simulink model "extra_blocks"  (Simulink 7.4)
settings: Solver=FixedStepDiscrete  StartTime=0.0  StopTime=10.0  RelTol=1e-3
undefined symbols (not defined in the file or in its folder): Ax, Ay, Az, DiscIntNeverNeededParam, lenA, sys1d, vargz
libraries: simulink x8, dspsigops x1, commanapbnd3 x1, instrumentlib x1
(part 1 of 2)
settings Model: Creator=iMose1  LastModifiedBy=iMose1

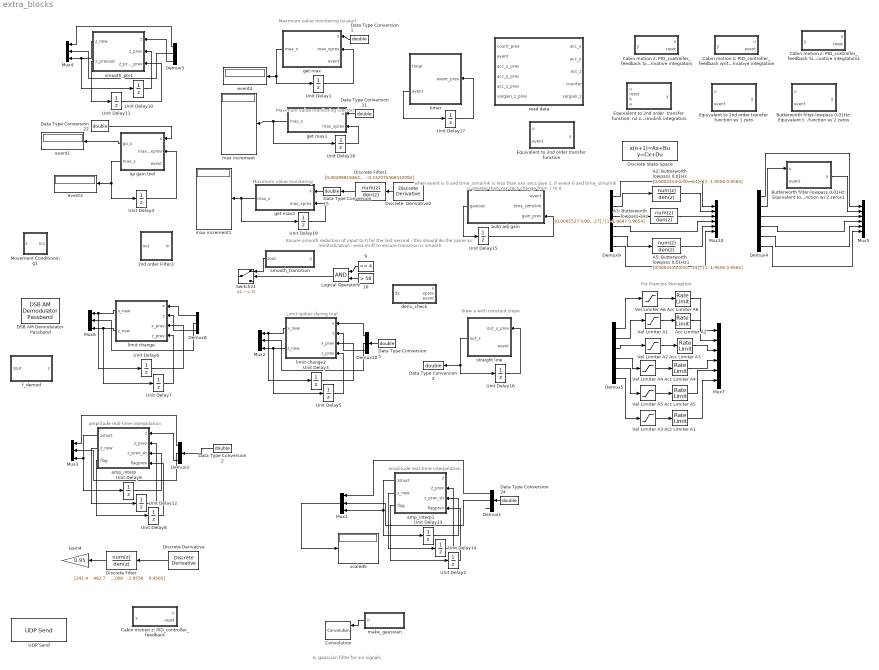
== system extra_blocks ==
  note: Limit spikes during trial
  note: amplitude real-time interpolation
  note: Ensure smooth reduction of input to 0
      | for the last second - this should do the
      | same as reinitialization - exta stuff
      | to ensure transition is smooth
  note: amplitude real-time interpolation
  note: draw a with
      | constant slope
  note: 6. gaussian filter
      | for sin signals
  note: when event is 6 and time_simulink is less than xxx secs give 1,
      | if event 6 and time_simulink is greater than xxx secs change from 1 to 0
  note: Maximum value monitoring (vector)
  note: Maximum value monitoring (scalar)
  note: Maximum value monitoring
  note: For Francois Perception
  "     10" : simulink/Logic and Bit Operations/Compare To Constant  SystemSampleTime=-1  relop=>  const=58  LogicOutDataTypeMode=uint8
  "     9" : simulink/Logic and Bit Operations/Compare To Constant  SystemSampleTime=-1  relop===  const=4  LogicOutDataTypeMode=uint8
  2nd order Filter2 : Subsystem
  A2: Butterworth lowpass 0.01Hz : DiscreteTransferFcn  Numerator=[0.0002414 0.0004827 0.0002414]  Denominator=[1 -1.9556 0.9565]  SampleTime=0.004
  A3: Butterworth lowpass 1Hz : DiscreteTransferFcn  Numerator=[0.0001527 0.0003054 0.0001527]  Denominator=[1 -1.9647 0.9654]  SampleTime=0.004
  A5: Butterworth lowpass 0.01Hz1 : DiscreteTransferFcn  Numerator=[0.0002414 0.0004827 0.0002414]  Denominator=[1 -1.9556 0.9565]  SampleTime=0.004
  Acc Limiter A1 : RateLimiter  RisingSlewLimit=0  FallingSlewLimit=0  SampleTimeMode=inherited
  Acc Limiter A2 : RateLimiter  RisingSlewLimit=0.05  FallingSlewLimit=-0.05  SampleTimeMode=inherited
  Acc Limiter A3 : RateLimiter  RisingSlewLimit=0.05  FallingSlewLimit=-0.05  SampleTimeMode=inherited
  Acc Limiter A4 : RateLimiter  RisingSlewLimit=0  FallingSlewLimit=0  SampleTimeMode=inherited
  Acc Limiter A5 : RateLimiter  RisingSlewLimit=0.05  FallingSlewLimit=-0.05  SampleTimeMode=inherited
  Acc Limiter A6 : RateLimiter  RisingSlewLimit=0  FallingSlewLimit=0  SampleTimeMode=inherited
  Butterworth filter-lowpass 0.01Hz: Equivalent to 2nd order transfer function w/ 2 zeros : Subsystem
  Butterworth filter-lowpass 0.01Hz: Equivalent to 2nd order transfer function w/ 2 zeros1 : Subsystem
  Cabin motion z: PID_controller_feedback : Subsystem
  Cabin motion z: PID_controller_feedback Simulink derivative integrators : Subsystem
  Cabin motion z: PID_controller_feedback Simulink derivative integrators1 : Subsystem
  Cabin motion z: PID_controller_feedback written derivative integration : Subsystem
  Convolution : dspsigops/Convolution  DialogController=dspDDGCreate  DialogControllerArgs=DataTag0  domain=Time  outputDataTypeStr=Inherit: Same as accumulator  outputLastDataTypeStr=Inherit: Same as accumulator  outputMin=[]  outputMax=[]  roundingMode=Floor  overflowMode=off
  DSB AM Demodulator Passband : commanapbnd3/DSB AM Demodulator Passband  SystemSampleTime=-1  Fc=0.091  Ph=0  method=Butterworth  n=4  cf=10  Rp=0.1  Rs=50  Offset=0
  Data Type Conversion{1..3,5,11,15,22,24} (8 alike) : DataTypeConversion  OutDataTypeMode=double  OutDataType=fixdt(1, 16)  OutScaling=2^0  OutDataTypeStr=double
  Demux{1..3,8,10} (5 alike) : Demux  Outputs=3
  Demux4 : Demux  Outputs=6
  Demux5 : Demux  Outputs=6
  Demux9 : Demux  Outputs=6
  Discrete  Derivative2 : simulink/Discrete/Discrete Derivative  SystemSampleTime=-1  gainval=1.0  ICPrevScaledInput=0.0  OutMin=[]  OutMax=[]  OutDataType=fixdt(1, 16)  OutScaling=2^-10  DoSatur=off
  Discrete Derivative : simulink/Discrete/Discrete Derivative  SystemSampleTime=-1  gainval=1.0  ICPrevScaledInput=0.0  OutMin=[]  OutMax=[]  OutDataType=fixdt(1, 16)  OutScaling=2^-10  DoSatur=off
  Discrete Filter : DiscreteFilter  Numerator="[241.4    482.7    241.4]"  Denominator="[1.0000   -1.9556    0.9565]"  SampleTime=0.004
  Discrete Filter1 : DiscreteFilter  Numerator="[0.002898194633721   0.008694583901164   0.008694583901164   0.002898194633721]"  Denominator="[1.000000000000000  -2.374094743709352   1.929355669091215  -0.532075368312092]"
  Discrete State-Space : DiscreteStateSpace  A=sys1d.a  B=sys1d.b  C=sys1d.c  D=sys1d.d  SampleTime=0.004
  Equivalent to 2nd order transfer function : Subsystem
  Equivalent to 2nd order transfer function w/ 1 zero : Subsystem
  "Equivalent to 2nd order  transfer function, no zeros, Simulink integrators" : Subsystem
  Gain4 : Gain  Gain=0.95  ParameterDataType=fixdt(1, 16)  ParameterScaling=2^0  OutDataType=fixdt(1, 16)  OutScaling=2^0
  Logical Operator9 : Logic  AllPortsSameDT=off  OutDataTypeMode=boolean  LogicDataType=fixdt(0, 8)  OutDataTypeStr=boolean
  Movement Conditioning1 : Subsystem
  Mux{1..4,6} (5 alike) : Mux  Inputs=3
  Mux10 : Mux  Inputs=6
  Mux5 : Mux  Inputs=6
  Mux7 : Mux  Inputs=6
  Switch21 : Switch  Criteria=u2 ~= 0  OutDataType=fixdt(1, 16)  OutScaling=2^0
  UDP Send : instrumentlib/UDP Send  DialogController=instrumentcreatedialog  DialogControllerArgs=DataTag1  Host='192.168.102.50'  Port=9800  LocalPort=-1  EnableBlockingMode=on  ByteOrder=BigEndian
  Unit Delay{1..17} (17 alike) : UnitDelay  SampleTime=-1
  Unit Delay18 : UnitDelay  X0=zeros(6,1)  SampleTime=-1
  Unit Delay19 : UnitDelay  X0=zeros(6,1)  SampleTime=-1
  Vel Limiter A1 : Saturate  UpperLimit=0.08  LowerLimit=-0.08  LinearizeAsGain=off  OutDataType=fixdt(1, 16)  OutScaling=2^0
  Vel Limiter A2 : Saturate  UpperLimit=0.05  LowerLimit=-0.05  OutDataType=fixdt(1, 16)  OutScaling=2^0
  Vel Limiter A3 : Saturate  UpperLimit=0  LowerLimit=0  OutDataType=fixdt(1, 16)  OutScaling=2^0
  Vel Limiter A4 : Saturate  UpperLimit=0  LowerLimit=0  OutDataType=fixdt(1, 16)  OutScaling=2^0
  Vel Limiter A5 : Saturate  UpperLimit=0.1  LowerLimit=-0.1  OutDataType=fixdt(1, 16)  OutScaling=2^0
  Vel Limiter A6 : Saturate  UpperLimit=0  LowerLimit=0  OutDataType=fixdt(1, 16)  OutScaling=2^0
  amp_interp : Stateflow chart
  amp_interp1 : Stateflow chart
  auto adj gain : Stateflow chart
  deriv_check : Stateflow chart
  event1 : Display
  event3 : Display
  event4 : Display
  f_demod : Stateflow chart
  get max : Stateflow chart
  get max1 : Stateflow chart
  get max2 : Stateflow chart
  limit change : Stateflow chart
  limit change2 : Stateflow chart
  make_gaussian : Stateflow chart
  max increment : Display
  max increment1 : Display
  op gain tool : Stateflow chart
  read data : Stateflow chart
  scaled5 : Display
  smooth_pts1 : Stateflow chart
  smooth_transition : Stateflow chart
  straight line : Stateflow chart
  timer : Subsystem
  wires:
  op gain tool/2(max_x) -> Unit Delay4/1, event3/1
  Unit Delay4/1 -> op gain tool/2(max_xprev)
  op gain tool/1(go_x) -> event1/1
  Data Type Conversion22/1 -> op gain tool/1(x)
  Demux8/1 -> limit change/1(x)
  Demux8/3 -> limit change/2(z)
  limit change/1(x_new) -> Mux6/1, Unit Delay6/1
  limit change/2(z_new) -> Mux6/3, Unit Delay7/1
  Demux8/2 -> Mux6/2
  Unit Delay6/1 -> limit change/3(x_prev)
  Unit Delay7/1 -> limit change/4(z_prev)
  Demux10/1 -> limit change2/1(x)
  Demux10/3 -> limit change2/2(z)
  limit change2/1(x_new) -> Mux2/1, Unit Delay3/1
  limit change2/2(z_new) -> Mux2/3, Unit Delay5/1
  Demux10/2 -> Mux2/2
  Unit Delay3/1 -> limit change2/3(x_prev)
  Unit Delay5/1 -> limit change2/4(z_prev)
  Data Type Conversion5/1 -> Demux10/1
  get max/1(max_x) -> Unit Delay1/1, event4/1
  Unit Delay1/1 -> get max/2(max_xprev)
  Data Type Conversion1/1 -> get max/1(x)
  Demux3/3 -> smooth_pts1/1(z)
  smooth_pts1/1(z_new) -> Mux4/3, Unit Delay10/1
  Demux3/2 -> Mux4/2
  Unit Delay10/1 -> smooth_pts1/2(z_prev)
  Demux3/1 -> Mux4/1
  smooth_pts1/2(z_prevout) -> Unit Delay11/1
  Unit Delay11/1 -> smooth_pts1/3(z_prev_prev)
  amp_interp/2(z_new) -> Unit Delay12/1
  Demux2/2 -> Mux3/2
  amp_interp/3(flag) -> Unit Delay8/1
  Unit Delay9/1 -> amp_interp/3(z_prev_sh)
  Demux2/1 -> Mux3/1
  amp_interp/1(zshort) -> Mux3/3, Unit Delay9/1
  Unit Delay12/1 -> amp_interp/2(z_prev)
  Unit Delay8/1 -> amp_interp/4(flagprev)
  Demux2/3 -> amp_interp/1(z)
  Data Type Conversion2/1 -> Demux2/1
  "     9"/1 -> Logical Operator9/1
  "     10"/1 -> Logical Operator9/2
  Logical Operator9/1 -> Switch21/2
  smooth_transition/1(zout) -> Switch21/1
  amp_interp1/2(z_new) -> Unit Delay14/1
  Demux1/2 -> Mux1/2
  Data Type Conversion24/1 -> Demux1/1
  amp_interp1/3(flag) -> Unit Delay2/1
  Unit Delay13/1 -> amp_interp1/3(z_prev_sh)
  Demux1/1 -> Mux1/1
  amp_interp1/1(zshort) -> Unit Delay13/1, Mux1/3
  Unit Delay14/1 -> amp_interp1/2(z_prev)
  Unit Delay2/1 -> amp_interp1/4(flagprev)
  Mux1/1 -> scaled5/1
  Demux1/3 -> ?
  ? -> amp_interp1/1(z)
  Discrete Derivative/1 -> Discrete Filter/1
  Discrete Filter/1 -> Gain4/1
  ? -> straight line/2(event)
  straight line/1(out_x) -> Unit Delay16/1, Data Type Conversion3/1
  Unit Delay16/1 -> straight line/1(out_x_prev)
  make_gaussian/1(h) -> Convolution/1
  auto adj gain/1(gainout) -> Unit Delay15/1
  Unit Delay15/1 -> auto adj gain/3(gain_prev)
  Unit Delay17/1 -> timer/1(event_prev)
  timer/2(event) -> Unit Delay17/1
  get max1/1(max_x) -> Unit Delay18/1, max increment/1
  Unit Delay18/1 -> get max1/2(max_xprev)
  Data Type Conversion11/1 -> get max1/1(x)
  Demux9/3 -> A3: Butterworth lowpass 1Hz/1
  Demux9/2 -> A2: Butterworth lowpass 0.01Hz/1
  Demux9/1 -> Mux10/1
  A2: Butterworth lowpass 0.01Hz/1 -> Mux10/2
  A3: Butterworth lowpass 1Hz/1 -> Mux10/3
  A5: Butterworth lowpass 0.01Hz1/1 -> Mux10/5
  Demux9/5 -> A5: Butterworth lowpass 0.01Hz1/1
  Demux9/6 -> Mux10/6
  Demux9/4 -> Mux10/4
  Demux4/3 -> Mux5/3
  Demux4/1 -> Mux5/1
  Butterworth filter-lowpass 0.01Hz: Equivalent to 2nd order transfer function w/ 2 zeros1/1(y) -> Mux5/2
  Demux4/5 -> Mux5/5
  Demux4/6 -> Mux5/6
  Demux4/4 -> Mux5/4
  Demux4/2 -> Butterworth filter-lowpass 0.01Hz: Equivalent to 2nd order transfer function w/ 2 zeros1/1(u)
  get max2/1(max_x) -> Unit Delay19/1, max increment1/1
  Unit Delay19/1 -> get max2/2(max_xprev)
  Data Type Conversion15/1 -> get max2/1(x)
  Discrete  Derivative2/1 -> Discrete Filter1/1
  Discrete Filter1/1 -> Data Type Conversion15/1
  Vel Limiter A1/1 -> Acc Limiter A2/1
  Vel Limiter A2/1 -> Acc Limiter A3/1
  Vel Limiter A5/1 -> Acc Limiter A5/1
  Demux5/5 -> Vel Limiter A5/1
  Acc Limiter A5/1 -> Mux7/5
  Acc Limiter A3/1 -> Mux7/3
  Demux5/3 -> Vel Limiter A2/1
  Acc Limiter A2/1 -> Mux7/2
  Demux5/2 -> Vel Limiter A1/1
  Vel Limiter A3/1 -> Acc Limiter A1/1
  Demux5/6 -> Vel Limiter A3/1
  Acc Limiter A1/1 -> Mux7/6
  Vel Limiter A4/1 -> Acc Limiter A4/1
  Demux5/4 -> Vel Limiter A4/1
  Acc Limiter A4/1 -> Mux7/4
  Vel Limiter A6/1 -> Acc Limiter A6/1
  Demux5/1 -> Vel Limiter A6/1
  Acc Limiter A6/1 -> Mux7/1

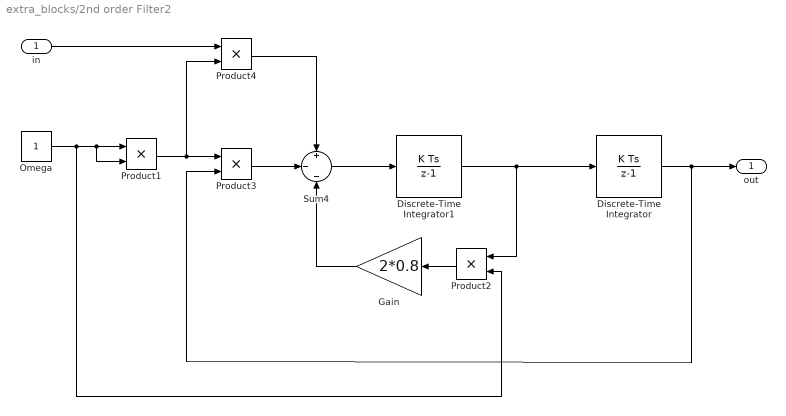
== system extra_blocks/2nd order Filter2 ==
  in : Inport
  Discrete-Time Integrator : DiscreteIntegrator  SampleTime=0.004  OutDataTypeMode=double  OutDataTypeStr=double  ICPrevOutput=DiscIntNeverNeededParam  ICPrevScaledInput=DiscIntNeverNeededParam
  Discrete-Time Integrator1 : DiscreteIntegrator  SampleTime=0.004  OutDataTypeMode=double  OutDataTypeStr=double  ICPrevOutput=DiscIntNeverNeededParam  ICPrevScaledInput=DiscIntNeverNeededParam
  Gain : Gain  Gain=2*0.8  ParameterDataType=fixdt(1, 16)  ParameterScaling=2^0  OutDataType=fixdt(1, 16)  OutScaling=2^0
  Omega : Constant  OutDataType=fixdt(1, 16)  OutScaling=2^0
  Product{1..4} (4 alike) : Product  RndMeth=Zero
  Sum4 : Sum  Inputs=+|-|-
  out : Outport
  wires:
  Omega/1 -> Product1/1, Product1/2, Product2/2
  Discrete-Time Integrator1/1 -> Discrete-Time Integrator/1, Product2/1
  Discrete-Time Integrator/1 -> out/1, Product3/2
  Sum4/1 -> Discrete-Time Integrator1/1
  Gain/1 -> Sum4/3
  Product2/1 -> Gain/1
  Product1/1 -> Product3/1, Product4/2
  Product3/1 -> Sum4/2
  in/1 -> Product4/1
  Product4/1 -> Sum4/1

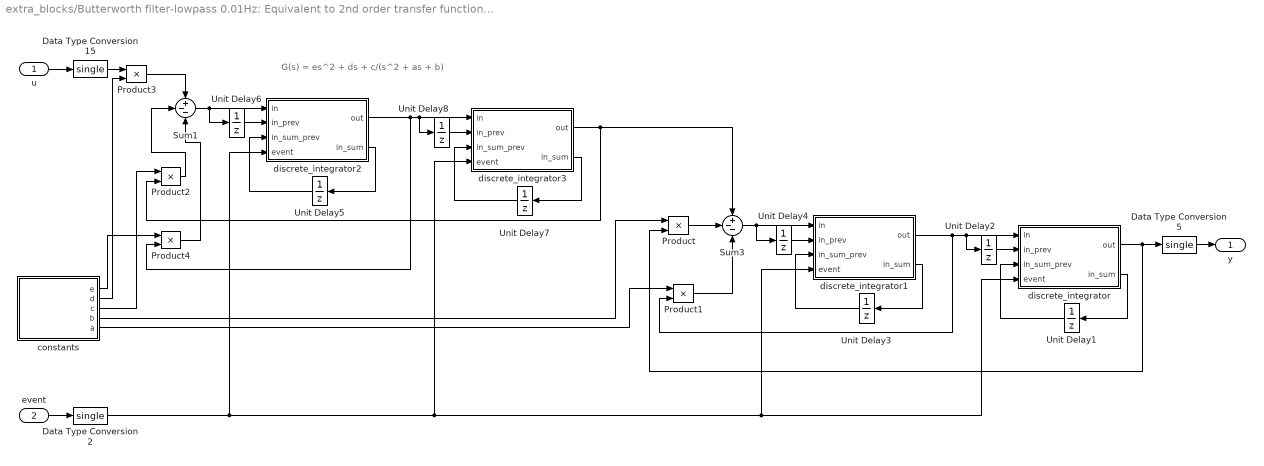
== system extra_blocks/Butterworth filter-lowpass 0.01Hz: Equivalent to 2nd order transfer function w/ 2 zeros ==
  note: G(s) = es^2 + ds + c/(s^2 + as + b)
  u : Inport
  event : Inport  Port=2
  Data Type Conversion15 : DataTypeConversion  OutDataTypeMode=single  OutDataType=fixdt(1, 16)  OutScaling=2^0  OutDataTypeStr=single
  Data Type Conversion2 : DataTypeConversion  OutDataTypeMode=single  OutDataType=fixdt(1, 16)  OutScaling=2^0  OutDataTypeStr=single
  Data Type Conversion5 : DataTypeConversion  OutDataTypeMode=single  OutDataType=fixdt(1, 16)  OutScaling=2^0  OutDataTypeStr=single
  Product{,1..4} (5 alike) : Product  OutDataType=fixdt(1, 16)  OutScaling=2^0  RndMeth=Zero
  Sum1 : Sum  Inputs=+--  OutDataType=fixdt(1, 16)  OutScaling=2^0
  Sum3 : Sum  Inputs=+--  OutDataType=fixdt(1, 16)  OutScaling=2^0
  Unit Delay{1..8} (8 alike) : UnitDelay  SampleTime=-1
  constants : Stateflow chart
  discrete_integrator : Stateflow chart
  discrete_integrator1 : Stateflow chart
  discrete_integrator2 : Stateflow chart
  discrete_integrator3 : Stateflow chart
  y : Outport
  wires:
  event/1 -> Data Type Conversion2/1
  Product/1 -> Sum3/2
  Product1/1 -> Sum3/3
  Data Type Conversion2/1 -> discrete_integrator2/4(event), discrete_integrator/4(event), discrete_integrator1/4(event), discrete_integrator3/4(event)
  discrete_integrator/1(out) -> Product/2, Data Type Conversion5/1
  discrete_integrator1/1(out) -> Product1/2, discrete_integrator/1(in), Unit Delay2/1
  Sum3/1 -> discrete_integrator1/1(in), Unit Delay4/1
  Data Type Conversion5/1 -> y/1
  constants/4(b) -> Product/1
  constants/5(a) -> Product1/1
  discrete_integrator2/1(out) -> discrete_integrator3/1(in), Unit Delay8/1, Product4/2
  constants/3(c) -> Product2/1
  Sum1/1 -> discrete_integrator2/1(in), Unit Delay6/1
  u/1 -> Data Type Conversion15/1
  Data Type Conversion15/1 -> Product3/1
  Product3/1 -> Sum1/1
  constants/2(d) -> Product3/2
  discrete_integrator/2(in_sum) -> Unit Delay1/1
  Unit Delay1/1 -> discrete_integrator/3(in_sum_prev)
  Unit Delay2/1 -> discrete_integrator/2(in_prev)
  discrete_integrator1/2(in_sum) -> Unit Delay3/1
  Unit Delay3/1 -> discrete_integrator1/3(in_sum_prev)
  Unit Delay4/1 -> discrete_integrator1/2(in_prev)
  discrete_integrator2/2(in_sum) -> Unit Delay5/1
  Unit Delay5/1 -> discrete_integrator2/3(in_sum_prev)
  Unit Delay6/1 -> discrete_integrator2/2(in_prev)
  discrete_integrator3/2(in_sum) -> Unit Delay7/1
  Unit Delay7/1 -> discrete_integrator3/3(in_sum_prev)
  Unit Delay8/1 -> discrete_integrator3/2(in_prev)
  discrete_integrator3/1(out) -> Sum3/1, Product2/2
  constants/1(e) -> Product4/1
  Product2/1 -> Sum1/2
  Product4/1 -> Sum1/3

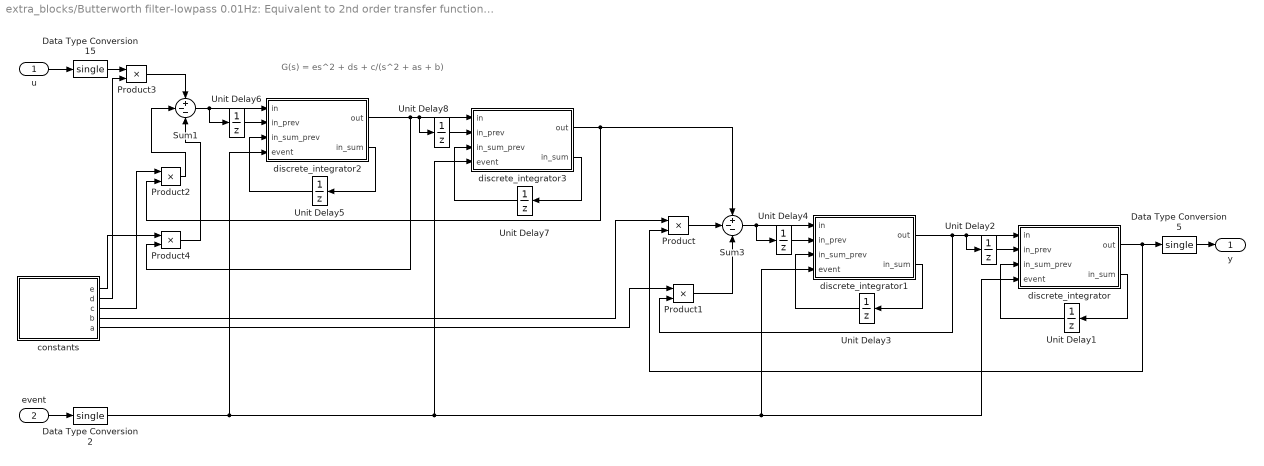
== system extra_blocks/Butterworth filter-lowpass 0.01Hz: Equivalent to 2nd order transfer function w/ 2 zeros1 ==
  note: G(s) = es^2 + ds + c/(s^2 + as + b)
  u : Inport
  event : Inport  Port=2
  Data Type Conversion15 : DataTypeConversion  OutDataTypeMode=single  OutDataType=fixdt(1, 16)  OutScaling=2^0  OutDataTypeStr=single
  Data Type Conversion2 : DataTypeConversion  OutDataTypeMode=single  OutDataType=fixdt(1, 16)  OutScaling=2^0  OutDataTypeStr=single
  Data Type Conversion5 : DataTypeConversion  OutDataTypeMode=single  OutDataType=fixdt(1, 16)  OutScaling=2^0  OutDataTypeStr=single
  Product{,1..4} (5 alike) : Product  OutDataType=fixdt(1, 16)  OutScaling=2^0  RndMeth=Zero
  Sum1 : Sum  Inputs=+--  OutDataType=fixdt(1, 16)  OutScaling=2^0
  Sum3 : Sum  Inputs=+--  OutDataType=fixdt(1, 16)  OutScaling=2^0
  Unit Delay{1..8} (8 alike) : UnitDelay  SampleTime=-1
  constants : Stateflow chart
  discrete_integrator : Stateflow chart
  discrete_integrator1 : Stateflow chart
  discrete_integrator2 : Stateflow chart
  discrete_integrator3 : Stateflow chart
  y : Outport
  wires:
  event/1 -> Data Type Conversion2/1
  Product/1 -> Sum3/2
  Product1/1 -> Sum3/3
  Data Type Conversion2/1 -> discrete_integrator2/4(event), discrete_integrator/4(event), discrete_integrator1/4(event), discrete_integrator3/4(event)
  discrete_integrator/1(out) -> Product/2, Data Type Conversion5/1
  discrete_integrator1/1(out) -> Product1/2, discrete_integrator/1(in), Unit Delay2/1
  Sum3/1 -> discrete_integrator1/1(in), Unit Delay4/1
  Data Type Conversion5/1 -> y/1
  constants/4(b) -> Product/1
  constants/5(a) -> Product1/1
  discrete_integrator2/1(out) -> discrete_integrator3/1(in), Unit Delay8/1, Product4/2
  constants/3(c) -> Product2/1
  Sum1/1 -> discrete_integrator2/1(in), Unit Delay6/1
  u/1 -> Data Type Conversion15/1
  Data Type Conversion15/1 -> Product3/1
  Product3/1 -> Sum1/1
  constants/2(d) -> Product3/2
  discrete_integrator/2(in_sum) -> Unit Delay1/1
  Unit Delay1/1 -> discrete_integrator/3(in_sum_prev)
  Unit Delay2/1 -> discrete_integrator/2(in_prev)
  discrete_integrator1/2(in_sum) -> Unit Delay3/1
  Unit Delay3/1 -> discrete_integrator1/3(in_sum_prev)
  Unit Delay4/1 -> discrete_integrator1/2(in_prev)
  discrete_integrator2/2(in_sum) -> Unit Delay5/1
  Unit Delay5/1 -> discrete_integrator2/3(in_sum_prev)
  Unit Delay6/1 -> discrete_integrator2/2(in_prev)
  discrete_integrator3/2(in_sum) -> Unit Delay7/1
  Unit Delay7/1 -> discrete_integrator3/3(in_sum_prev)
  Unit Delay8/1 -> discrete_integrator3/2(in_prev)
  discrete_integrator3/1(out) -> Sum3/1, Product2/2
  constants/1(e) -> Product4/1
  Product2/1 -> Sum1/2
  Product4/1 -> Sum1/3

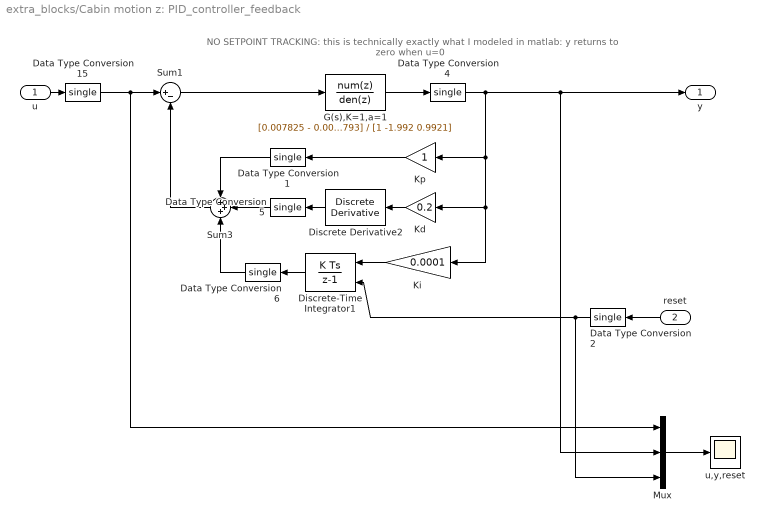
== system extra_blocks/Cabin motion z: PID_controller_feedback ==
  note: NO SETPOINT TRACKING: this is technically exactly what I modeled in matlab:
      | y returns to zero when u=0
  u : Inport
  reset : Inport  Port=2
  Data Type Conversion{1..2,4..6,15} (6 alike) : DataTypeConversion  OutDataTypeMode=single  OutDataType=fixdt(1, 16)  OutScaling=2^0  OutDataTypeStr=single
  Discrete Derivative2 : simulink/Discrete/Discrete Derivative  SystemSampleTime=-1  gainval=1.0  ICPrevScaledInput=0.0  OutMin=[]  OutMax=[]  OutDataType=fixdt(1, 16)  OutScaling=2^-10  DoSatur=off
  Discrete-Time Integrator1 : DiscreteIntegrator  ExternalReset=rising  SampleTime=0.004  OutDataType=fixdt(1, 16)  OutScaling=2^0  ICPrevOutput=DiscIntNeverNeededParam  ICPrevScaledInput=DiscIntNeverNeededParam
  G(s),K=1,a=1 : DiscreteTransferFcn  Numerator=[0.007825 - 0.007793]  Denominator=[1 -1.992 0.9921]  SampleTime=0.004
  Kd : Gain  Gain=0.2  ParameterDataType=fixdt(1, 16)  ParameterScaling=2^0  OutDataType=fixdt(1, 16)  OutScaling=2^0
  Ki : Gain  Gain=0.0001  ParameterDataType=fixdt(1, 16)  ParameterScaling=2^0  OutDataType=fixdt(1, 16)  OutScaling=2^0
  Kp : Gain  ParameterDataType=fixdt(1, 16)  ParameterScaling=2^0  OutDataType=fixdt(1, 16)  OutScaling=2^0
  Mux : Mux  Inputs=3
  Sum1 : Sum  Inputs=|+-  OutDataType=fixdt(1, 16)  OutScaling=2^0
  Sum3 : Sum  Inputs=+++  OutDataType=fixdt(1, 16)  OutScaling=2^0
  u,y,reset : Scope
      settings: YMin=-1  YMax=1
  y : Outport
  wires:
  Kd/1 -> Discrete Derivative2/1
  Ki/1 -> Discrete-Time Integrator1/1
  Kp/1 -> Data Type Conversion1/1
  Discrete Derivative2/1 -> Data Type Conversion5/1
  Discrete-Time Integrator1/1 -> Data Type Conversion6/1
  reset/1 -> Data Type Conversion2/1
  u/1 -> Data Type Conversion15/1
  Sum1/1 -> G(s),K=1,a=1/1
  G(s),K=1,a=1/1 -> Data Type Conversion4/1
  Sum3/1 -> Sum1/2
  Mux/1 -> u,y,reset/1
  Data Type Conversion15/1 -> Sum1/1, Mux/1
  Data Type Conversion4/1 -> Ki/1, Kd/1, Kp/1, y/1, Mux/2
  Data Type Conversion1/1 -> Sum3/1
  Data Type Conversion5/1 -> Sum3/2
  Data Type Conversion6/1 -> Sum3/3
  Data Type Conversion2/1 -> Discrete-Time Integrator1/2, Mux/3

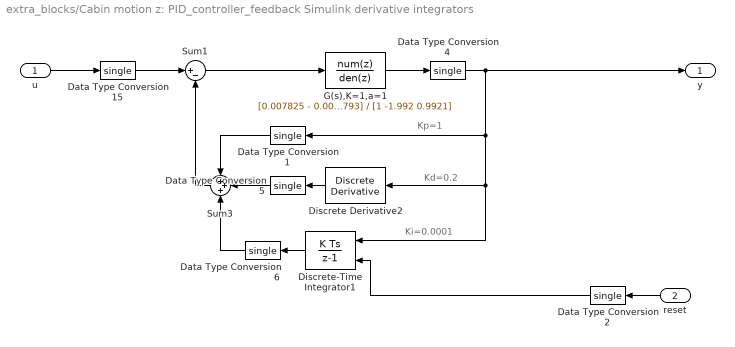
== system extra_blocks/Cabin motion z: PID_controller_feedback Simulink derivative integrators ==
  note: Kp=1
  note: Kd=0.2
  note: Ki=0.0001
  u : Inport
  reset : Inport  Port=2
  Data Type Conversion{1..2,4..6,15} (6 alike) : DataTypeConversion  OutDataTypeMode=single  OutDataType=fixdt(1, 16)  OutScaling=2^0  OutDataTypeStr=single
  Discrete Derivative2 : simulink/Discrete/Discrete Derivative  SystemSampleTime=-1  gainval=0.2  ICPrevScaledInput=0.0  OutMin=[]  OutMax=[]  OutDataType=fixdt(1, 16)  OutScaling=2^-10  DoSatur=off
  Discrete-Time Integrator1 : DiscreteIntegrator  gainval=0.0001  ExternalReset=rising  SampleTime=0.004  OutDataType=fixdt(1, 16)  OutScaling=2^0  ICPrevOutput=DiscIntNeverNeededParam  ICPrevScaledInput=DiscIntNeverNeededParam
  G(s),K=1,a=1 : DiscreteTransferFcn  Numerator=[0.007825 - 0.007793]  Denominator=[1 -1.992 0.9921]  SampleTime=0.004
  Sum1 : Sum  Inputs=|+-  OutDataType=fixdt(1, 16)  OutScaling=2^0
  Sum3 : Sum  Inputs=+++  OutDataType=fixdt(1, 16)  OutScaling=2^0
  y : Outport
  wires:
  Discrete Derivative2/1 -> Data Type Conversion5/1
  Discrete-Time Integrator1/1 -> Data Type Conversion6/1
  reset/1 -> Data Type Conversion2/1
  u/1 -> Data Type Conversion15/1
  Sum1/1 -> G(s),K=1,a=1/1
  G(s),K=1,a=1/1 -> Data Type Conversion4/1
  Sum3/1 -> Sum1/2
  Data Type Conversion15/1 -> Sum1/1
  Data Type Conversion4/1 -> Discrete Derivative2/1, Discrete-Time Integrator1/1, Data Type Conversion1/1, y/1
  Data Type Conversion1/1 -> Sum3/1
  Data Type Conversion5/1 -> Sum3/2
  Data Type Conversion6/1 -> Sum3/3
  Data Type Conversion2/1 -> Discrete-Time Integrator1/2

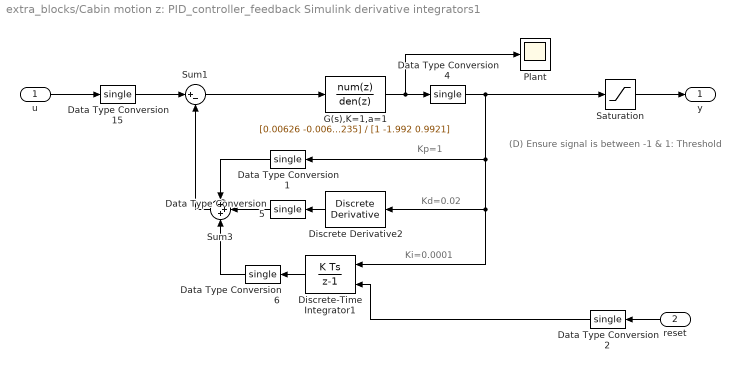
== system extra_blocks/Cabin motion z: PID_controller_feedback Simulink derivative integrators1 ==
  note: Kp=1
  note: Kd=0.02
  note: Ki=0.0001
  note: (D) Ensure signal
      | is between -1 & 1:
      | Threshold
  u : Inport
  reset : Inport  Port=2
  Data Type Conversion{1..2,4..6,15} (6 alike) : DataTypeConversion  OutDataTypeMode=single  OutDataType=fixdt(1, 16)  OutScaling=2^0  OutDataTypeStr=single
  Discrete Derivative2 : simulink/Discrete/Discrete Derivative  SystemSampleTime=-1  gainval=0.02  ICPrevScaledInput=0.0  OutMin=[]  OutMax=[]  OutDataType=fixdt(1, 16)  OutScaling=2^-10  DoSatur=off
  Discrete-Time Integrator1 : DiscreteIntegrator  gainval=0.0001  ExternalReset=rising  SampleTime=0.004  OutDataType=fixdt(1, 16)  OutScaling=2^0  ICPrevOutput=DiscIntNeverNeededParam  ICPrevScaledInput=DiscIntNeverNeededParam
  G(s),K=1,a=1 : DiscreteTransferFcn  Numerator=[0.00626 -0.006235]  Denominator=[1 -1.992 0.9921]  SampleTime=0.004
  Plant : Scope
      settings: TimeRange=100  YMin=-1  YMax=1  SaveName=ScopeData2
  Saturation : Saturate  UpperLimit=0.3  LowerLimit=-0.3  OutDataType=fixdt(1, 16)  OutScaling=2^0
  Sum1 : Sum  Inputs=|+-  OutDataType=fixdt(1, 16)  OutScaling=2^0
  Sum3 : Sum  Inputs=+++  OutDataType=fixdt(1, 16)  OutScaling=2^0
  y : Outport
  wires:
  Discrete Derivative2/1 -> Data Type Conversion5/1
  Discrete-Time Integrator1/1 -> Data Type Conversion6/1
  reset/1 -> Data Type Conversion2/1
  u/1 -> Data Type Conversion15/1
  Sum1/1 -> G(s),K=1,a=1/1
  G(s),K=1,a=1/1 -> Data Type Conversion4/1, Plant/1
  Sum3/1 -> Sum1/2
  Data Type Conversion15/1 -> Sum1/1
  Data Type Conversion4/1 -> Discrete Derivative2/1, Discrete-Time Integrator1/1, Data Type Conversion1/1, Saturation/1
  Data Type Conversion1/1 -> Sum3/1
  Data Type Conversion5/1 -> Sum3/2
  Data Type Conversion6/1 -> Sum3/3
  Data Type Conversion2/1 -> Discrete-Time Integrator1/2
  Saturation/1 -> y/1

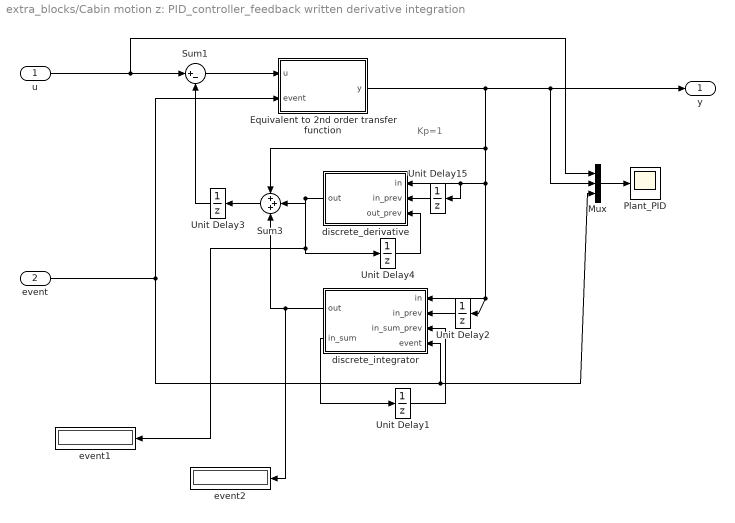
== system extra_blocks/Cabin motion z: PID_controller_feedback written derivative integration ==
  note: Kp=1
  u : Inport
  event : Inport  Port=2
  Equivalent to 2nd order transfer function : Subsystem
  Mux : Mux  Inputs=3
  Plant_PID : Scope
  Sum1 : Sum  Inputs=|+-  OutDataType=fixdt(1, 16)  OutScaling=2^0
  Sum3 : Sum  Inputs=+++  OutDataType=fixdt(1, 16)  OutScaling=2^0
  Unit Delay{1..4,15} (5 alike) : UnitDelay  SampleTime=-1
  discrete_derivative : Stateflow chart
  discrete_integrator : Stateflow chart
  event1 : Display
  event2 : Display
  y : Outport
  wires:
  event/1 -> Equivalent to 2nd order transfer function/2(event), discrete_integrator/4(event), Mux/3
  u/1 -> Sum1/1, Mux/1
  Sum3/1 -> Unit Delay3/1
  Sum1/1 -> Equivalent to 2nd order transfer function/1(u)
  Equivalent to 2nd order transfer function/1(y) -> discrete_integrator/1(in), Unit Delay2/1, discrete_derivative/1(in), Unit Delay15/1, Sum3/1, y/1, Mux/2
  discrete_derivative/1(out) -> Sum3/2, Unit Delay4/1, event1/1
  discrete_integrator/1(out) -> Sum3/3, event2/1
  discrete_integrator/2(in_sum) -> Unit Delay1/1
  Unit Delay1/1 -> discrete_integrator/3(in_sum_prev)
  Unit Delay2/1 -> discrete_integrator/2(in_prev)
  Unit Delay15/1 -> discrete_derivative/2(in_prev)
  Unit Delay3/1 -> Sum1/2
  Unit Delay4/1 -> discrete_derivative/3(out_prev)
  Mux/1 -> Plant_PID/1

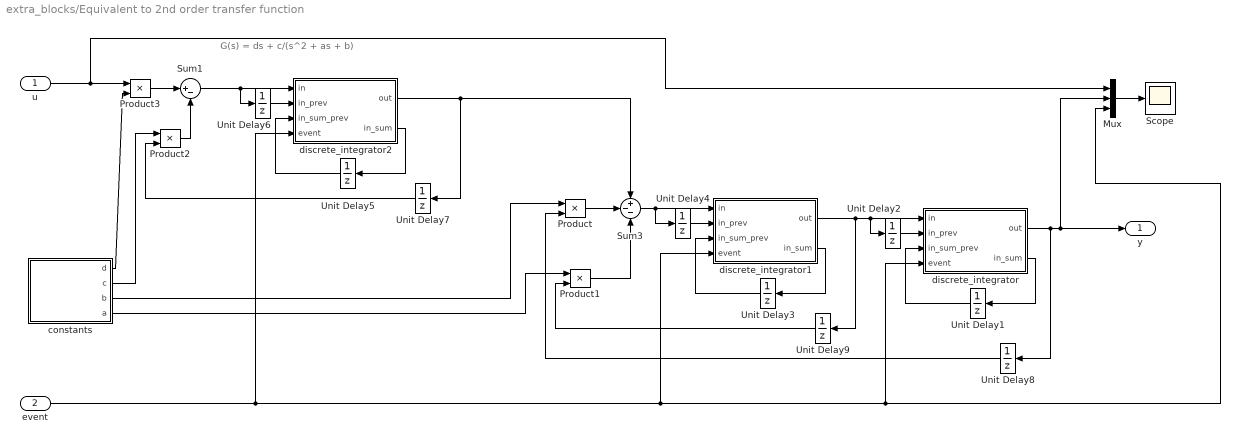
== system extra_blocks/Equivalent to 2nd order transfer function ==
  note: G(s) = ds + c/(s^2 + as + b)
  u : Inport
  event : Inport  Port=2
  Mux : Mux  Inputs=3
  Product{,1..3} (4 alike) : Product  OutDataType=fixdt(1, 16)  OutScaling=2^0  RndMeth=Zero
  Scope : Scope
      settings: TimeRange=60  YMin=-1.75  YMax=4
  Sum1 : Sum  Inputs=|+-  OutDataType=fixdt(1, 16)  OutScaling=2^0
  Sum3 : Sum  Inputs=+--  OutDataType=fixdt(1, 16)  OutScaling=2^0
  Unit Delay{1..9} (9 alike) : UnitDelay  SampleTime=-1
  constants : Stateflow chart
  discrete_integrator : Stateflow chart
  discrete_integrator1 : Stateflow chart
  discrete_integrator2 : Stateflow chart
  y : Outport
  wires:
  event/1 -> discrete_integrator1/4(event), discrete_integrator/4(event), Mux/3, discrete_integrator2/4(event)
  Product/1 -> Sum3/2
  Product1/1 -> Sum3/3
  discrete_integrator/1(out) -> Unit Delay8/1, y/1, Mux/2
  discrete_integrator1/1(out) -> discrete_integrator/1(in), Unit Delay2/1, Unit Delay9/1
  Sum3/1 -> discrete_integrator1/1(in), Unit Delay4/1
  constants/3(b) -> Product/1
  constants/4(a) -> Product1/1
  constants/2(c) -> Product2/1
  Product2/1 -> Sum1/2
  u/1 -> Product3/1, Mux/1
  Product3/1 -> Sum1/1
  constants/1(d) -> Product3/2
  discrete_integrator/2(in_sum) -> Unit Delay1/1
  Unit Delay1/1 -> discrete_integrator/3(in_sum_prev)
  Unit Delay2/1 -> discrete_integrator/2(in_prev)
  discrete_integrator1/2(in_sum) -> Unit Delay3/1
  Unit Delay3/1 -> discrete_integrator1/3(in_sum_prev)
  Unit Delay4/1 -> discrete_integrator1/2(in_prev)
  discrete_integrator2/2(in_sum) -> Unit Delay5/1
  Unit Delay5/1 -> discrete_integrator2/3(in_sum_prev)
  Unit Delay6/1 -> discrete_integrator2/2(in_prev)
  Unit Delay8/1 -> Product/2
  Unit Delay9/1 -> Product1/2
  Unit Delay7/1 -> Product2/2
  Mux/1 -> Scope/1
  discrete_integrator2/1(out) -> Sum3/1, Unit Delay7/1
  Sum1/1 -> discrete_integrator2/1(in), Unit Delay6/1

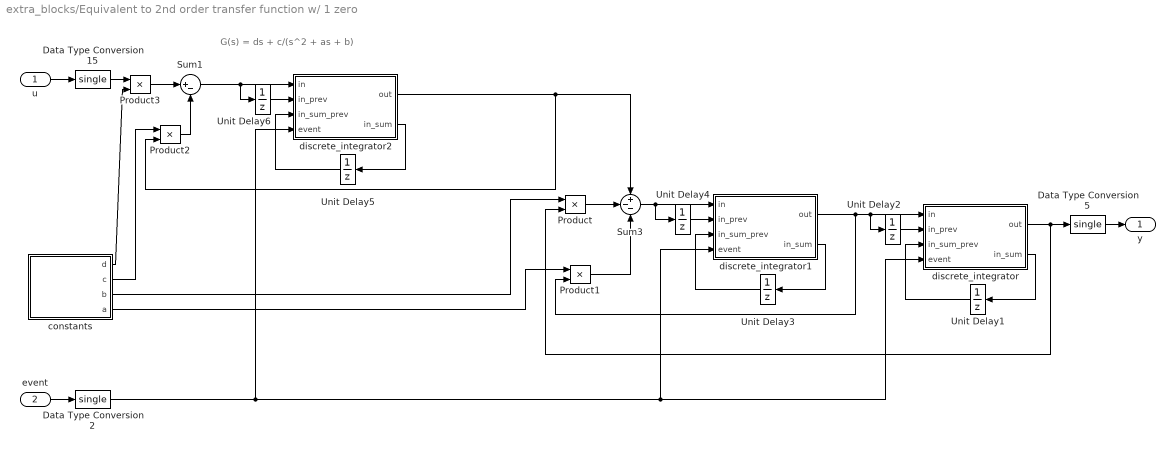
== system extra_blocks/Equivalent to 2nd order transfer function w/ 1 zero ==
  note: G(s) = ds + c/(s^2 + as + b)
  u : Inport
  event : Inport  Port=2
  Data Type Conversion15 : DataTypeConversion  OutDataTypeMode=single  OutDataType=fixdt(1, 16)  OutScaling=2^0  OutDataTypeStr=single
  Data Type Conversion2 : DataTypeConversion  OutDataTypeMode=single  OutDataType=fixdt(1, 16)  OutScaling=2^0  OutDataTypeStr=single
  Data Type Conversion5 : DataTypeConversion  OutDataTypeMode=single  OutDataType=fixdt(1, 16)  OutScaling=2^0  OutDataTypeStr=single
  Product{,1..3} (4 alike) : Product  OutDataType=fixdt(1, 16)  OutScaling=2^0  RndMeth=Zero
  Sum1 : Sum  Inputs=|+-  OutDataType=fixdt(1, 16)  OutScaling=2^0
  Sum3 : Sum  Inputs=+--  OutDataType=fixdt(1, 16)  OutScaling=2^0
  Unit Delay{1..6} (6 alike) : UnitDelay  SampleTime=-1
  constants : Stateflow chart
  discrete_integrator : Stateflow chart
  discrete_integrator1 : Stateflow chart
  discrete_integrator2 : Stateflow chart
  y : Outport
  wires:
  event/1 -> Data Type Conversion2/1
  Product/1 -> Sum3/2
  Product1/1 -> Sum3/3
  Data Type Conversion2/1 -> discrete_integrator/4(event), discrete_integrator1/4(event), discrete_integrator2/4(event)
  discrete_integrator/1(out) -> Product/2, Data Type Conversion5/1
  discrete_integrator1/1(out) -> Product1/2, discrete_integrator/1(in), Unit Delay2/1
  Sum3/1 -> discrete_integrator1/1(in), Unit Delay4/1
  Data Type Conversion5/1 -> y/1
  constants/3(b) -> Product/1
  constants/4(a) -> Product1/1
  discrete_integrator2/1(out) -> Product2/2, Sum3/1
  constants/2(c) -> Product2/1
  Product2/1 -> Sum1/2
  Sum1/1 -> discrete_integrator2/1(in), Unit Delay6/1
  u/1 -> Data Type Conversion15/1
  Data Type Conversion15/1 -> Product3/1
  Product3/1 -> Sum1/1
  constants/1(d) -> Product3/2
  discrete_integrator/2(in_sum) -> Unit Delay1/1
  Unit Delay1/1 -> discrete_integrator/3(in_sum_prev)
  Unit Delay2/1 -> discrete_integrator/2(in_prev)
  discrete_integrator1/2(in_sum) -> Unit Delay3/1
  Unit Delay3/1 -> discrete_integrator1/3(in_sum_prev)
  Unit Delay4/1 -> discrete_integrator1/2(in_prev)
  discrete_integrator2/2(in_sum) -> Unit Delay5/1
  Unit Delay5/1 -> discrete_integrator2/3(in_sum_prev)
  Unit Delay6/1 -> discrete_integrator2/2(in_prev)

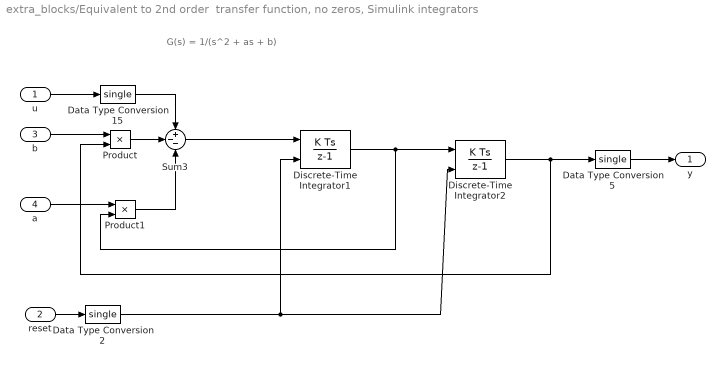
== system extra_blocks/Equivalent to 2nd order  transfer function, no zeros, Simulink integrators ==
  note: G(s) = 1/(s^2 + as + b)
  u : Inport
  reset : Inport  Port=2
  b : Inport  Port=3
  a : Inport  Port=4
  Data Type Conversion15 : DataTypeConversion  OutDataTypeMode=single  OutDataType=fixdt(1, 16)  OutScaling=2^0  OutDataTypeStr=single
  Data Type Conversion2 : DataTypeConversion  OutDataTypeMode=single  OutDataType=fixdt(1, 16)  OutScaling=2^0  OutDataTypeStr=single
  Data Type Conversion5 : DataTypeConversion  OutDataTypeMode=single  OutDataType=fixdt(1, 16)  OutScaling=2^0  OutDataTypeStr=single
  Discrete-Time Integrator1 : DiscreteIntegrator  gainval=1  ExternalReset=rising  SampleTime=0.004  OutDataType=fixdt(1, 16)  OutScaling=2^0  ICPrevOutput=DiscIntNeverNeededParam  ICPrevScaledInput=DiscIntNeverNeededParam
  Discrete-Time Integrator2 : DiscreteIntegrator  gainval=1  ExternalReset=rising  SampleTime=0.004  OutDataType=fixdt(1, 16)  OutScaling=2^0  ICPrevOutput=DiscIntNeverNeededParam  ICPrevScaledInput=DiscIntNeverNeededParam
  Product : Product  OutDataType=fixdt(1, 16)  OutScaling=2^0  RndMeth=Zero
  Product1 : Product  OutDataType=fixdt(1, 16)  OutScaling=2^0  RndMeth=Zero
  Sum3 : Sum  Inputs=+--  OutDataType=fixdt(1, 16)  OutScaling=2^0
  y : Outport
  wires:
  reset/1 -> Data Type Conversion2/1
  u/1 -> Data Type Conversion15/1
  Data Type Conversion15/1 -> Sum3/1
  Product/1 -> Sum3/2
  Product1/1 -> Sum3/3
  Data Type Conversion2/1 -> Discrete-Time Integrator1/2, Discrete-Time Integrator2/2
  Discrete-Time Integrator2/1 -> Product/2, Data Type Conversion5/1
  Discrete-Time Integrator1/1 -> Discrete-Time Integrator2/1, Product1/2
  Sum3/1 -> Discrete-Time Integrator1/1
  b/1 -> Product/1
  a/1 -> Product1/1
  Data Type Conversion5/1 -> y/1

== system extra_blocks/Movement Conditioning1 ==
  note: Position
      | x,y,z for iMose
  note: Position
      | unity
  note: coordinate frame Unity -> iMose
  note: His unity signal is 0 during non-trial,
      | but during the trial it starts at 91.  Make
      | the trial values start at 0 (by adding -91),
      | and make the non-trial values at 0 too.
  In1 : Inport
  Compare To Constant2 : simulink/Logic and Bit Operations/Compare To Constant  SystemSampleTime=-1  relop=~=  const=0  LogicOutDataTypeMode=uint8
  Constant3 : Constant  Value=-91  OutDataType=fixdt(1, 16)  OutScaling=2^0
  Data Type Conversion11 : DataTypeConversion  OutDataTypeMode=single  OutDataType=fixdt(1, 16)  OutScaling=2^0  OutDataTypeStr=single
  Demux1 : Demux  Outputs=3
  Gain : Gain  Gain=-1  ParameterDataType=fixdt(1, 16)  ParameterScaling=2^0  OutDataType=fixdt(1, 16)  OutScaling=2^0
  Mux1 : Mux  Inputs=3
  Sum7 : Sum  Inputs=++|  OutDataType=fixdt(1, 16)  OutScaling=2^0
  Switch21 : Switch  Criteria=u2 ~= 0  OutDataType=fixdt(1, 16)  OutScaling=2^0
  Out1 : Outport
  wires:
  In1/1 -> Demux1/1
  Demux1/3 -> Mux1/1
  Demux1/1 -> Mux1/2
  Data Type Conversion11/1 -> Gain/1
  Mux1/1 -> Out1/1
  Compare To Constant2/1 -> Switch21/2
  Gain/1 -> Mux1/3
  Demux1/2 -> Compare To Constant2/1, Sum7/2, Switch21/3
  Sum7/1 -> Switch21/1
  Constant3/1 -> Sum7/1
  Switch21/1 -> Data Type Conversion11/1

== system extra_blocks/timer ==
  event_prev : Inport  OutDataType=fixdt(1, 16)  OutScaling=2^0
  Clock1 : Clock
      settings: Decimation=10
  Unit Delay10 : UnitDelay  SampleTime=-1
  Unit Delay9 : UnitDelay  SampleTime=-1
  read data : Stateflow chart
  timer : Outport
  event : Outport  Port=2
  wires:
  read data/4(timer) -> timer/1
  read data/1(event) -> event/1
  read data/2(trial_rest_flag) -> Unit Delay10/1
  Unit Delay10/1 -> read data/2(trial_rest_flag_prev)
  event_prev/1 -> read data/1(event_prev)
  Clock1/1 -> read data/3(clock_new)
  Unit Delay9/1 -> read data/4(clock_start_prev)
  read data/3(clock_start) -> Unit Delay9/1

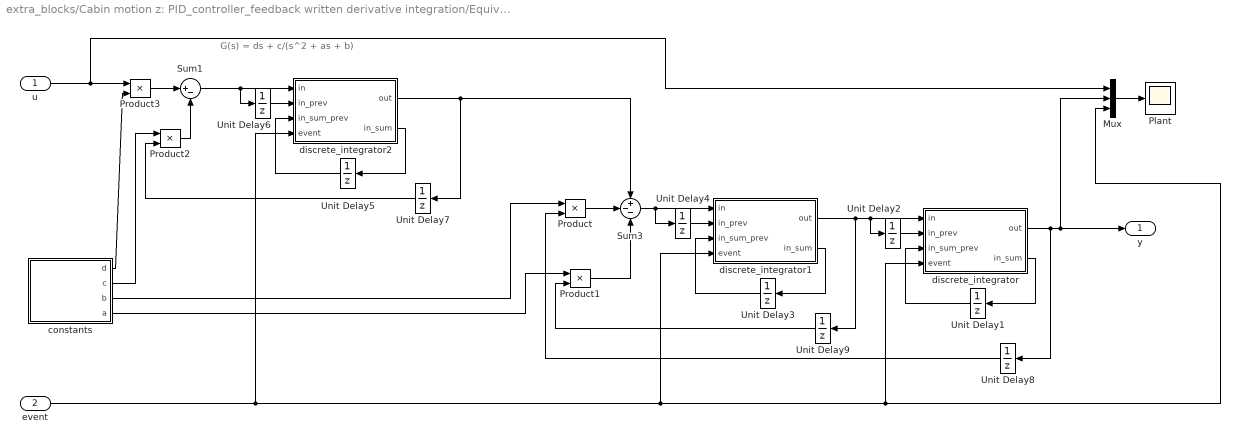
== system extra_blocks/Cabin motion z: PID_controller_feedback written derivative integration/Equivalent to 2nd order transfer function ==
  note: G(s) = ds + c/(s^2 + as + b)
  u : Inport
  event : Inport  Port=2
  Mux : Mux  Inputs=3
  Plant : Scope
      settings: TimeRange=60  YMin=-1.75  YMax=4
  Product{,1..3} (4 alike) : Product  OutDataType=fixdt(1, 16)  OutScaling=2^0  RndMeth=Zero
  Sum1 : Sum  Inputs=|+-  OutDataType=fixdt(1, 16)  OutScaling=2^0
  Sum3 : Sum  Inputs=+--  OutDataType=fixdt(1, 16)  OutScaling=2^0
  Unit Delay{1..9} (9 alike) : UnitDelay  SampleTime=-1
  constants : Stateflow chart
  discrete_integrator : Stateflow chart
  discrete_integrator1 : Stateflow chart
  discrete_integrator2 : Stateflow chart
  y : Outport
  wires:
  event/1 -> discrete_integrator1/4(event), discrete_integrator/4(event), Mux/3, discrete_integrator2/4(event)
  Product/1 -> Sum3/2
  Product1/1 -> Sum3/3
  discrete_integrator/1(out) -> Unit Delay8/1, y/1, Mux/2
  discrete_integrator1/1(out) -> discrete_integrator/1(in), Unit Delay2/1, Unit Delay9/1
  Sum3/1 -> discrete_integrator1/1(in), Unit Delay4/1
  constants/3(b) -> Product/1
  constants/4(a) -> Product1/1
  constants/2(c) -> Product2/1
  Product2/1 -> Sum1/2
  u/1 -> Product3/1, Mux/1
  Product3/1 -> Sum1/1
  constants/1(d) -> Product3/2
  discrete_integrator/2(in_sum) -> Unit Delay1/1
  Unit Delay1/1 -> discrete_integrator/3(in_sum_prev)
  Unit Delay2/1 -> discrete_integrator/2(in_prev)
  discrete_integrator1/2(in_sum) -> Unit Delay3/1
  Unit Delay3/1 -> discrete_integrator1/3(in_sum_prev)
  Unit Delay4/1 -> discrete_integrator1/2(in_prev)
  discrete_integrator2/2(in_sum) -> Unit Delay5/1
  Unit Delay5/1 -> discrete_integrator2/3(in_sum_prev)
  Unit Delay6/1 -> discrete_integrator2/2(in_prev)
  Unit Delay8/1 -> Product/2
  Unit Delay9/1 -> Product1/2
  Unit Delay7/1 -> Product2/2
  Mux/1 -> Plant/1
  discrete_integrator2/1(out) -> Sum3/1, Unit Delay7/1
  Sum1/1 -> discrete_integrator2/1(in), Unit Delay6/1

== matlab function smooth_transition ==
  data: z input double; zout output double
function zout = ampin(z)

%#eml

max_inc = 0.01;

if z == 0
    zout = z;
else
    if z > 0
        zout = z - max_inc;
    else
        %z < 0
        zout = z + max_inc;
    end
end

== matlab function get max ==
  data: x input double; max_x output double; max_xprev input double; event input double
function max_x = f(x, max_xprev, event)

%#eml
if (event == 3) || (event == 4)

    max_x = max(abs(x)); % want max deviation from 0

    if max_x < max_xprev
        max_x = max_xprev;
    end
else
    max_x = 0;
end

== matlab function op gain tool ==
  data: x input double; go_x output double; max_xprev input double; max_x output double; event input double
function [go_x, max_x] = ggo(x, max_xprev, event)

%#eml
% Get Gain Optimal (ggo):
% Tool for iMose: finding the gain that maximizes the range of movement for iMose without causing a stop.

% Before, finding the optimal gain values for x,y,z was done by trial-and-error.  But this takes a lot of time.



max_x = max(abs(x)); % want max deviation from 0

if max_x < max_xprev
    max_x = max_xprev;
end


% It would be good to put a timer here, to wait for 5 seconds before
% evaluating the max_x value; wait for some data to be collected.


opt_value = 1;  % the maximum input value that iMose can do is if the value is around 1 (ie: 1)
buffer = 0.25;

if max_x < (opt_value/3)  % Values are really low
    max_range = opt_value/3;
    go_x = 1/max_range - buffer;
else
    if (opt_value/3) < max_x < ((2*opt_value)/3)
        max_range = (2*opt_value)/3;
        go_x = 1/max_range - buffer;
    else
        go_x = buffer;
    end
end

== matlab function amp_interp ==
  data: z input double; z_prev input double; z_prev_sh input double; zshort output double; flagprev input double; z_new output double; flag output double
function [zshort, z_new, flag] = ampin(z, z_prev, z_prev_sh, flagprev)

%#eml

max_inc = 0.1;
%max_inc = 0.0039;

z_new = z;
%if abs(z) ~= abs(z_prev)
if abs(z-z_prev) > max_inc
    if z > z_prev
        if flagprev == 1
            zshort = z_prev + max_inc;
        else
            zshort = z_prev_sh + max_inc;
        end
    else
        if flagprev == 1
            zshort = z_prev - max_inc;
        else
            zshort = z_prev_sh - max_inc;
        end
    end
    flag = 0;
else
    zshort = z;
    flag = 1;
end

== matlab function smooth_pts1 ==
  data: z input double; z_prev input double; z_new output double; z_prev_prev input double; z_prevout output double
function [z_new, z_prevout] = smooth_pts(z, z_prev, z_prev_prev)
%#eml

n = 3;

z_prevout = z_prev;

z_new = (z + z_prev + z_prev_prev)/n;

== matlab function amp_interp1 ==
  data: z input double; z_prev input double; z_prev_sh input double; zshort output double; flagprev input double; z_new output double; flag output double
function [zshort, z_new, flag] = ampin(z, z_prev, z_prev_sh, flagprev)

%#eml

max_inc = 0.1;
%max_inc = 0.0039;

z_new = z;

if abs(z-z_prev) > max_inc
    if z > z_prev
        if flagprev == 1
            zshort = z_prev + max_inc;
        else
            zshort = z_prev_sh + max_inc;
        end
    else
        if flagprev == 1
            zshort = z_prev - max_inc;
        else
            zshort = z_prev_sh - max_inc;
        end
    end
    flag = 0;
else
    if flagprev == 1
        zshort = z;
        flag = 1;
    else
        zshort = z_prev_sh;  % important: when there are no jumps in the signal it needs to continue tracing the "short" curve
        flag = 0;
    end
end

== matlab function f_demod ==
  data: z input double; zout output double
function zout = demod(z)

eml.extrinsic('amdemod');

Fs = 252;
Fc = 0.091;
zout = 4.1*amdemod(z, Fc, Fs);

== matlab function read data ==
  data: Ax parameter double; Ay parameter double; Az parameter double; lenA parameter double; vargz parameter double; acc_x output double; acc_y output double; acc_z output double; count_prev input double; event input double; counter output double; acc_x_prev input double; acc_y_prev input double; acc_z_prev input double; vargain_z_prev input double; vargain_z output double
function [acc_x, acc_y, acc_z, counter, vargain_z] = strmdat(Ax, Ay, Az, lenA, vargz, count_prev, event, ...
    acc_x_prev, acc_y_prev, acc_z_prev, vargain_z_prev)
%#eml


acc_x = acc_x_prev;
acc_y = acc_y_prev;
acc_z = acc_z_prev;
vargain_z = vargain_z_prev;

counter = count_prev;


if (event == 3 || event == 4) && (count_prev <= (lenA-1))  % trial 3 and 4 is running and not at the end of the defined data 
    counter = count_prev + 1;
    
    acc_x = Ax(counter, 1);
    acc_y = Ay(counter, 1);
    acc_z = -Az(counter, 1);
    vargain_z = vargz(counter, 1);
else
    counter = 0;   % reset counter
    acc_x = 0;
    acc_y = 0;
    acc_z = 0;
    vargain_z = 0;
end

== matlab function timer/read data ==
  data: event output double; trial_rest_flag output double; clock_start output double; timer output double; event_prev input double; trial_rest_flag_prev input double; clock_new input double; clock_start_prev input double
function [event, trial_rest_flag, clock_start, timer] = ...
    f(event_prev, trial_rest_flag_prev, clock_new, clock_start_prev)

%#eml
restlen = 0.1;   % max length period in seconds

% ------------------------------------------------------------
% Method 2: based on a timer, determine when the time is finished
% ------------------------------------------------------------
current_clock = clock_new;
clock_start = clock_start_prev;

timer = (current_clock - clock_start);  % was output to keep track of time per event

event = event_prev;
trial_rest_flag = trial_rest_flag_prev;

if event == 0   % Event = 0: EXP started (Pushed Connect_X)
    event = 1;  % Event = 1: Read new line in trial matrix
    
    trial_rest_flag = 2;
    clock_start = clock_new;  % Compute how long it takes to load a new trial
else
    if (event == 1)
        
        % Rest and Trial: count up trial, read new line of trial matrix
        event = 2;  % Event 2: Rest count only
        
        trial_rest_flag = 1;  % 1 = rest, 2 = trial1, 3 = trial2, 4 = finished trial and reading a new line
        clock_start = clock_new;  % for REST
        timer = 0;
    else
        
        % Determine if we are in Rest, Trial1, Trial2, Reinitialization
        switch trial_rest_flag 
            case 1  % REST period count
                % Check trcou to see if the alotted trial time is finished
                if (current_clock - clock_start) > restlen
                    event = 1;
                    trial_rest_flag = 1;
                    clock_start = clock_new;
                    timer = 0;
                else
                    % Rest period count is NOT finished - reasigned the same values
                    clock_start = clock_start_prev; % hold the initial clock value for REST
                end
                
        end  % end of switch trial_rest_flag
        
    end
end

== matlab function get max1 ==
  data: x input double; max_x output double; max_xprev input double
function max_x  = f(x, max_xprev)

%#eml

%if (event > 1)

    max_x1 = max(abs(x(1,1))); % want max deviation from 0
    if max_x1 < max_xprev(1,1)
        max_x1 = max_xprev(1,1);
    end
    
    max_x2 = max(abs(x(2,1))); % want max deviation from 0
    if max_x2 < max_xprev(2,1)
        max_x2 = max_xprev(2,1);
    end
    
    max_x3 = max(abs(x(3,1))); % want max deviation from 0
    if max_x3 < max_xprev(3,1)
        max_x3 = max_xprev(3,1);
    end
    
    max_x4 = max(abs(x(4,1))); % want max deviation from 0
    if max_x4 < max_xprev(4,1)
        max_x4 = max_xprev(4,1);
    end
    
    max_x5 = max(abs(x(5,1))); % want max deviation from 0
    if max_x5 < max_xprev(5,1)
        max_x5 = max_xprev(5,1);
    end
    
    max_x6 = max(abs(x(6,1))); % want max deviation from 0
    if max_x6 < max_xprev(6,1)
        max_x6 = max_xprev(6,1);
    end
    
% else
%     max_x1 = 0;
%     max_x2 = 0;
%     max_x3 = 0;
%     max_x4 = 0;
%     max_x5 = 0;
%     max_x6 = 0;
% end

max_x = [max_x1; max_x2; max_x3; max_x4; max_x5; max_x6];

== matlab function limit change ==
  data: x input double; z input double; x_new output double; x_prev input double; z_prev input double; z_new output double
function [x_new, z_new] = limchange(x, z, x_prev, z_prev)
%#eml

max_inc = 0.3;
%max_inc = 0.0039;

if abs(x - x_prev) > max_inc
    x_new = max_inc + x;
else
    x_new = x;
end

if abs(z - z_prev) > max_inc
    z_new = max_inc + z;
else
    z_new = z;
end

== matlab function Cabin motion z: PID_controller_feedback written derivative integration/discrete_derivative ==
  data: out output double; in input double; in_prev input double; out_prev input double
function out = f(in, in_prev, out_prev)

%#eml

Kd = 0.0002;

% Performs the discrete derivative
dt = 0.004;

if (isnan(in_prev) == 1) || (isnan(in) == 1) || (isinf(in_prev) == 1) || (isinf(in) == 1)
    out = out_prev;
else
    temp = Kd*((in-in_prev)/dt);
    if (isnan(temp) == 1) || (isinf(temp) == 1)
        out = out_prev;
    else
        out = temp;
    end
end

== matlab function limit change2 ==
  data: x input double; z input double; x_new output double; x_prev input double; z_prev input double; z_new output double
function [x_new, z_new] = limchange(x, z, x_prev, z_prev)
%#eml

% Limit spikes during and at the end of the trial

max_inc = 0.05;
%max_inc = 0.0039;

if abs(x) ~= abs(x_prev)
    if abs(x - x_prev) > max_inc
        x_new = max_inc;  % error: x_new = max_inc + x;
    else
        x_new = x;
    end
else
    %if abs(x) == 1
        % means current and previous values are equal - this can happen when value exceeds acceleration limit and I set the acceleration at 1
        % Meaning: the input value is a spike or is huge
        %x_new = x/10 + max_inc;  % make output small and increase by max_inc - it will increase by 0.1 instead of 1
    %else
        x_new = max_inc;
    %end
end


if abs(z) ~= abs(z_prev)
    if abs(z - z_prev) > max_inc
        z_new = max_inc;
    else
        z_new = z;
    end
else
    % means current and previous values are equal - this can happen when value exceeds acceleration limit and I set the acceleration at 1
    z_new = max_inc;
end

== matlab function Cabin motion z: PID_controller_feedback written derivative integration/Equivalent to 2nd order transfer function/constants ==
  data: d output double; c output double; b output double; a output double
function [d, c, b, a] = f

%#eml

% Plant: G(s) = ds + c/(s^2 + as + b)

% -----------------------
% zeta = sqrt(2)/2;
% om = 1.4;   % from 1.4 to 1.0
% K = 1;
% a = 1;  % small

% num = [K*(om^2)/a K*om^2];   % (om^2/a)(s+a)
% den = [1 2*zeta*om om^2];
% sysout = tf(num, den);

% num = [0.007825 - 0.007793]
% den = [1 -1.992 0.9921]

% Transfer function:     (K=1,a=1 - iMose can do this plant)
% 0.007825 z - 0.007793
% ----------------------
% z^2 - 1.992 z + 0.9921
% -------> large response signal
% -----------------------

% -----------------------
% zeta = sqrt(2)/2;
% om = 1.4;   % from 1.4 to 1.0
% K = 0.5;
% a = 1;  % small
% num = [K*(om^2)/a K*om^2];   % (om^2/a)(s+a)
% den = [1 2*zeta*om om^2];
% sysout = tf(num, den);
% Ts = 0.004;
% c2d(sysout, Ts)

% Transfer function:
% 0.003912 z - 0.003897
% ----------------------
% z^2 - 1.992 z + 0.9921
%  
% Sampling time: 0.004
% -----------------------


% Discrete coefficients
b = 0.09921;
a = -0.1992;
c = -0.4793;
d = 0.4825;

== matlab function deriv_check ==
  data: x input double; dx output double; xprev input double; event input double
function dx = nder(x, xprev, event)

%#eml
% scalar value

ts = 0.004;
if event == 4
    dx = (x - xprev)/ts;
else
    dx = 0;
end

== matlab function make_gaussian ==
  data: h output double
function h = f

%#eml
eml.extrinsic('gaussfir');

BT = 0.004; % BT product --> B=3-dB bandwidth * T (input signal's period) 
OF = 50;  % Number of samples per symbol (N) --> Oversampling factor
NT = 50;  % Group delay (number of symbols) --> 2 symbol periods to the filters peak. 
filtgain = 3600;   % Linear amplitude filter gain
h = filtgain*gaussfir(BT,NT,OF);

== matlab function auto adj gain ==
  data: event input double; gainout output double; time_simulink input double; gain_prev input double
function gainout = fcn(event, time_simulink, gain_prev)

%#eml

% If free flight is  3mins(180secs) start auto-tune gain 10secs before end
% Test: free flight is 1min (60secs) start auto-tune gain 10secs before end
max_ff = 60; 
time_to_decrease = 10;  % sec

if (event == 6) && (time_simulink < (max_ff - time_to_decrease))
    gainout = 1;
else
    % Do slow stop
    num_of_iter = (time_to_decrease)/0.004;
    gainout = gain_prev - 1/num_of_iter;
end

== matlab function Cabin motion z: PID_controller_feedback written derivative integration/discrete_integrator ==
  data: out output double; in input double; in_prev input double; in_sum_prev input double; in_sum output double; event input double
function [out, in_sum] = f(in, in_prev, in_sum_prev, event)

%#eml

Ki = 0.0001;

if (event == 4)
    % Sum the input
    in_increment = in - in_prev;
    in_sum = in_sum_prev + in_increment;
    out = Ki*(in_sum);
else
    % Reset
    in_sum = 0;
    out = 0;
end

== matlab function straight line ==
  data: out_x_prev input double; out_x output double; event input double
function out_x = line(out_x_prev, event)
%#eml

rate_inc  = 3.1356/600;  % slope

if (event ~= 4)
    out_x = 0;
else
    out_x = rate_inc + out_x_prev;  % keep moving straight   
end

== matlab function Cabin motion z: PID_controller_feedback written derivative integration/Equivalent to 2nd order transfer function/discrete_integrator ==
  data: out output double; in input double; in_prev input double; in_sum_prev input double; in_sum output double; event input double
function [out, in_sum] = f(in, in_prev, in_sum_prev, event)

%#eml

Ki = 1;

if (event == 4)
    % Sum the input
    in_increment = in - in_prev;
    in_sum = in_sum_prev + in_increment;
    out = Ki*(in_sum);
else
    % Reset
    in_sum = 0;
    out = 0;
end

== matlab function Cabin motion z: PID_controller_feedback written derivative integration/Equivalent to 2nd order transfer function/discrete_integrator1 ==
  data: out output double; in input double; in_prev input double; in_sum_prev input double; in_sum output double; event input double
function [out, in_sum] = f(in, in_prev, in_sum_prev, event)

%#eml

Ki = 1;

if (event == 4)
    % Sum the input
    in_increment = in - in_prev;
    in_sum = in_sum_prev + in_increment;
    out = Ki*(in_sum);
else
    % Reset
    in_sum = 0;
    out = 0;
end

== matlab function Cabin motion z: PID_controller_feedback written derivative integration/Equivalent to 2nd order transfer function/discrete_integrator2 ==
  data: out output double; in input double; in_prev input double; in_sum_prev input double; in_sum output double; event input double
function [out, in_sum] = f(in, in_prev, in_sum_prev, event)

%#eml

Ki = 1;

if (event == 4)
    % Sum the input
    in_increment = in - in_prev;
    in_sum = in_sum_prev + in_increment;
    out = Ki*(in_sum);
else
    % Reset
    in_sum = 0;
    out = 0;
end
